simulink library "carnot"  (R2013b)
settings: Solver=ode45  StartTime=0.0  StopTime=10.0  RelTol=1e-3
undefined symbols (not defined in the file or in its folder): A, acol, Ahabit, Awin, Azimuth_Angle, AziWin, B, C, c1, c4, capc, caph, CarnotCallbacks_Density, CarnotCallbacks_Enthalpy, CarnotCallbacks_Enthalpy2Temperature, CarnotCallbacks_Entropy, CarnotCallbacks_Evaporation_Enthalpy, CarnotCallbacks_GlobalMessageLevel, CarnotCallbacks_Grashof, CarnotCallbacks_Heat_Capacity, CarnotCallbacks_Kinematic_Viscosity, CarnotCallbacks_Prandtl, CarnotCallbacks_Saturation_Property, CarnotCallbacks_Saturation_Temperature, CarnotCallbacks_Saturation_Value_Water, CarnotCallbacks_Specific_Volume, CarnotCallbacks_Thermal_Conductivity, CarnotCallbacks_Vapour_Content, CarnotCallbacks_Vapour_Pressure, con, cond, d, Dd, density, dfin, dia, DiameterLastPiece, DPConstant, dpipe, DPLinear, DPQuadratic, emission_out, fluid, FluidMix, FluidType, FPC, frame, g, GeodeticHeight, Gwin, heat_capacity, hgt, HP, Hroom, ID, inlet, K, l, lin, lpipe ... (+29)
undefined symbols (not defined in the file): c2, c3, c5, c6, cwall, dactive, height, mc, mID, rho, tau, UAneighbour, UAwall, uloss
libraries: carnot x333, simulink x25, simulink_extras x7
(part 10 of 16)

== system carnot/Basic/Thermal_Models/sfun_storage_heatexchanger ==
  Tnodes : Inport
  THBin : Inport  Port=2
  Bus Selector : BusSelector  OutputSignals=Temperature,MassFlow,Pressure,FluidType,FluidMix
  Mux1 : Mux  Inputs=5
  storeHX : S-Function  FunctionName=storage_heatexchanger  Parameters=id, nodes, inlet, outlet, pp(1), pp(2), pp(3), pp(4), pp(5), pp(6), pp(7)  EnableBusSupport=off
  Qnodes : Outport
  Thx : Outport  Port=2
  wires:
  Mux1/1 -> storeHX/2
  Bus Selector/5 -> Mux1/5  "<FluidMix>"
  Bus Selector/4 -> Mux1/4  "<FluidType>"
  Bus Selector/3 -> Mux1/3  "<Pressure>"
  Bus Selector/2 -> Mux1/2  "<MassFlow>"
  Bus Selector/1 -> Mux1/1  "<Temperature>"
  Tnodes/1 -> storeHX/1
  storeHX/1 -> Qnodes/1
  THBin/1 -> Bus Selector/1
  storeHX/2 -> Thx/1

== system carnot/Basic/Ventilation/Window_Ventilation ==
  Troom : Inport
  Tamb : Inport  Port=2
  control : Inport  Port=3
  Mux : Mux  Inputs=3
  S-Function : S-Function  FunctionName=tiltvent  Parameters=alpha, H, W  EnableBusSupport=off
  V_rate [m^3/s] : Outport
  wires:
  Tamb/1 -> Mux/2
  control/1 -> Mux/3
  S-Function/1 -> V_rate [m^3/s]/1
  Mux/1 -> S-Function/1
  Troom/1 -> Mux/1

== system carnot/Basic/Weather_and_Sun/Cloudage ==
  Iglob : Inport
  S : Constant  Value=latitude
  S-Function : S-Function  FunctionName=metcloud_s  Parameters=skytype  EnableBusSupport=off
  S1 : Constant  Value=longitude
  S2 : Constant  Value=longitude0
  mux5 : Mux
  cloudage : Outport
  wires:
  S1/1 -> mux5/3
  S/1 -> mux5/2
  mux5/1 -> S-Function/1
  S2/1 -> mux5/4
  S-Function/1 -> cloudage/1
  Iglob/1 -> mux5/1

== system carnot/Basic/Weather_and_Sun/Radiation_Divison ==
  Iglob : Inport
  Demux5 : Demux  Outputs=5
  S : Constant  Value=latitude
  S-Function : S-Function  FunctionName=metrad_s  EnableBusSupport=off
  S1 : Constant  Value=longitude
  S2 : Constant  Value=longitude0
  mux5 : Mux
  Idir : Outport
  Idfu : Outport  Port=2
  SunAngle : Outport  Port=3
  Zenith : Outport  Port=4
  Azimuth : Outport  Port=5
  wires:
  Demux5/5 -> Azimuth/1
  Demux5/4 -> Zenith/1
  Demux5/3 -> SunAngle/1
  Demux5/2 -> Idfu/1
  Demux5/1 -> Idir/1
  S-Function/1 -> Demux5/1
  mux5/1 -> S-Function/1
  Iglob/1 -> mux5/1
  S/1 -> mux5/2
  S1/1 -> mux5/3
  S2/1 -> mux5/4

== system carnot/Basic/Weather_and_Sun/Sky_Temperature ==
  Tamb : Inport
  hum : Inport  Port=2
  cloudage : Inport  Port=3
  S-Function : S-Function  FunctionName=metsky_s  Parameters=tskymodel  EnableBusSupport=off
  mux6 : Mux  Inputs=3
  Tsky : Outport
  wires:
  S-Function/1 -> Tsky/1
  mux6/1 -> S-Function/1
  Tamb/1 -> mux6/1
  hum/1 -> mux6/2
  cloudage/1 -> mux6/3

== system carnot/Basic/Weather_and_Sun/Solar_Declination_Angle ==
  time : Inport
  S-Function : S-Function  FunctionName=solardeclination  EnableBusSupport=off
  declination : Outport
  wires:
  time/1 -> S-Function/1
  S-Function/1 -> declination/1

== system carnot/Basic/Weather_and_Sun/Solar_Extraterrestrial_Radiation ==
  time : Inport
  S-Function : S-Function  FunctionName=solarextraterrestrialradiaton  EnableBusSupport=off
  I_extra : Outport
  wires:
  S-Function/1 -> I_extra/1
  time/1 -> S-Function/1

== system carnot/Basic/Weather_and_Sun/Solar_Hour_Angle ==
  note: hourangle = (true_solar_time - 12*3600)*2*pi/24/3600
  time : Inport
  2*pi/(24*3600) : Gain  Gain=2*pi/(24*3600)
  Add : Sum  Inputs=+-
  Constant : Constant  Value=12*3600
  S-Function : S-Function  FunctionName=solartime  Parameters=timezone, longitude  EnableBusSupport=off
  solar_hour_angle : Outport
  wires:
  time/1 -> S-Function/1
  S-Function/1 -> Add/1
  Add/1 -> 2*pi/(24*3600)/1
  2*pi/(24*3600)/1 -> solar_hour_angle/1
  Constant/1 -> Add/2

== system carnot/Basic/Weather_and_Sun/Solar_Position ==
  Solar_Position : S-Function  FunctionName=sunpos  Parameters=longi lati timezone  EnableBusSupport=off
  Out1 : Outport
  wires:
  Solar_Position/1 -> Out1/1

== system carnot/Basic/Weather_and_Sun/Solar_Time ==
  time : Inport
  S-Function : S-Function  FunctionName=solartime  Parameters=timezone, longitude  EnableBusSupport=off
  solartime : Outport
  wires:
  S-Function/1 -> solartime/1
  time/1 -> S-Function/1

== system carnot/Basic/Weather_and_Sun/WDB_Creator ==
  TimeValueComment : Inport
  Zenith_Angle : Inport  Port=2
  Azimuth_Angle : Inport  Port=3
  Solar_Radiation_beam_normal : Inport  Port=4
  Solar_Radiation_diffuse_horizontal : Inport  Port=5
  Temperature_Ambient : Inport  Port=6
  Temperature_Sky_Radiation : Inport  Port=7
  Relative_Humidity : Inport  Port=8
  Precipitation : Inport  Port=9
  Cloud_Index : Inport  Port=10
  Station_Pressure : Inport  Port=11
  Wind_Speed : Inport  Port=12
  Wind_Direction : Inport  Port=13
  Incidence_Angle_sun : Inport  Port=14
  Incidence_Angle_longitudinal : Inport  Port=15
  Incidence_Angle_transversal : Inport  Port=16
  Solar_Radiation_direct_surface : Inport  Port=17
  Solar_Radiation_diffuse_surface : Inport  Port=18
  Bus Creator : BusCreator  InitFcn=load WDB.mat  Inputs=18  OutDataTypeStr=Bus: WDB
  WDB : Outport
  wires:
  Bus Creator/1 -> WDB/1  "WDB"
  Solar_Radiation_diffuse_surface/1 -> Bus Creator/18  "Solar_Radiation_diffuse_surface"
  Solar_Radiation_direct_surface/1 -> Bus Creator/17  "Solar_Radiation_direct_surface"
  Incidence_Angle_transversal/1 -> Bus Creator/16  "Incidence_Angle_transversal"
  Incidence_Angle_longitudinal/1 -> Bus Creator/15  "Incidence_Angle_longitudinal"
  Incidence_Angle_sun/1 -> Bus Creator/14  "Incidence_Angle_sun"
  Wind_Direction/1 -> Bus Creator/13  "Wind_Direction"
  Wind_Speed/1 -> Bus Creator/12  "Wind_Speed"
  Station_Pressure/1 -> Bus Creator/11  "Station_Pressure"
  Cloud_Index/1 -> Bus Creator/10  "Cloud_Index"
  Precipitation/1 -> Bus Creator/9  "Precipitation"
  Relative_Humidity/1 -> Bus Creator/8  "Relative_Humidity"
  Temperature_Sky_Radiation/1 -> Bus Creator/7  "Temperature_Sky_Radiation"
  Temperature_Ambient/1 -> Bus Creator/6  "Temperature_Ambient"
  Solar_Radiation_diffuse_horizontal/1 -> Bus Creator/5  "Solar_Radiation_diffuse_horizontal"
  Azimuth_Angle/1 -> Bus Creator/3  "Azimuth_Angle"
  Zenith_Angle/1 -> Bus Creator/2  "Zenith_Angle"
  TimeValueComment/1 -> Bus Creator/1  "TimeValueComment"
  Solar_Radiation_beam_normal/1 -> Bus Creator/4  "Solar_Radiation_beam_normal"

== system carnot/Hydraulics/Flow_Diverter/Subsystem ==
  In1 : Inport
  Bus Selector10 : BusSelector  OutputSignals=MassFlow,DPConstant,DPLinear,DPQuadratic
  Mux : Mux
  Out1 : Outport
  wires:
  Mux/1 -> Out1/1
  In1/1 -> Bus Selector10/1
  Bus Selector10/4 -> Mux/4  "<DPQuadratic>"
  Bus Selector10/3 -> Mux/3  "<DPLinear>"
  Bus Selector10/2 -> Mux/2  "<DPConstant>"
  Bus Selector10/1 -> Mux/1  "<MassFlow>"

== system carnot/Hydraulics/Flow_Diverter/increase_ID ==
  In1 : Inport
  Abs : Abs
  Bias : Bias  Bias=1
  Dot Product1 : DotProduct  InputSameDT=on  OutDataTypeStr=Inherit: Inherit via internal rule
  Sign : Signum
  Out1 : Outport
  wires:
  In1/1 -> Abs/1, Sign/1
  Dot Product1/1 -> Out1/1
  Abs/1 -> Bias/1
  Sign/1 -> Dot Product1/1
  Bias/1 -> Dot Product1/2

== system carnot/Hydraulics/Flow_Mixer/PT1_for_fdiv ==
  ID_1 : Inport
  ID_2 : Inport  Port=2
  fdiv : Inport  Port=3
  Compare To Zero : simulink/Logic and Bit Operations/Compare To Zero  relop=<=  OutDataTypeStr=uint8
  Compare To Zero1 : simulink/Logic and Bit Operations/Compare To Zero  relop=<=  OutDataTypeStr=uint8
  Constant : Constant  Value=0
  Constant1 : Constant
  Gain1 : Gain  Gain=2
  Index Vector : MultiPortSwitch  DataPortOrder=Zero-based contiguous  zeroidx=on
  MinMax2 : MinMax  Function=max  Inputs=2
  Transfer Fcn (with initial states) : simulink_extras/Additional Linear/Transfer Fcn (with initial states)  N=[1]  D="[t  1]"  X0=0.5
  f_div : Outport
  wires:
  Index Vector/1 -> f_div/1
  Gain1/1 -> MinMax2/2
  Constant1/1 -> Index Vector/4
  Transfer Fcn (with initial states)/1 -> Index Vector/2
  Constant/1 -> Index Vector/3
  ID_2/1 -> Compare To Zero1/1
  ID_1/1 -> Compare To Zero/1
  MinMax2/1 -> Index Vector/1
  Compare To Zero/1 -> MinMax2/1
  Compare To Zero1/1 -> Gain1/1
  fdiv/1 -> Transfer Fcn (with initial states)/1

== system carnot/Hydraulics/Flow_Mixer_Thermostatic/Icontrol_fdiv ==
  ID_1 : Inport
  ID_2 : Inport  Port=2
  Twarm : Inport  Port=3
  Tset : Inport  Port=4
  Compare To Zero : simulink/Logic and Bit Operations/Compare To Zero  relop=<=  OutDataTypeStr=uint8
  Compare To Zero1 : simulink/Logic and Bit Operations/Compare To Zero  relop=<=  OutDataTypeStr=uint8
  Constant : Constant  Value=0
  Constant1 : Constant
  Gain : Gain  Gain=t1  SaturateOnIntegerOverflow=on  OutDataTypeStr=Inherit: Same as input  ParamDataTypeStr=Inherit: Same as input
  Gain1 : Gain  Gain=2
  Index Vector : MultiPortSwitch  DataPortOrder=Zero-based contiguous  zeroidx=on
  Integrator : Integrator  LimitOutput=on  UpperSaturationLimit=1  LowerSaturationLimit=0
  MinMax2 : MinMax  Function=max  Inputs=2
  diff_T : Sum  Inputs=-+  SaturateOnIntegerOverflow=on  InputSameDT=on  OutDataTypeStr=Inherit: Same as first input
  f_div : Outport
  wires:
  diff_T/1 -> Gain/1
  Gain/1 -> Integrator/1
  Twarm/1 -> diff_T/1
  Tset/1 -> diff_T/2
  Index Vector/1 -> f_div/1
  Gain1/1 -> MinMax2/2
  Constant1/1 -> Index Vector/4
  Integrator/1 -> Index Vector/2
  Constant/1 -> Index Vector/3
  ID_2/1 -> Compare To Zero1/1
  ID_1/1 -> Compare To Zero/1
  MinMax2/1 -> Index Vector/1
  Compare To Zero/1 -> MinMax2/1
  Compare To Zero1/1 -> Gain1/1

== system carnot/Hydraulics/Valve_ThermoTset/thermostat charcteristic ==
  T : Inport
  Tset : Inport  Port=2
  Backlash : Backlash  BacklashWidth=bl
  Bias : Bias  Bias=op
  Bias1 : Bias  Bias=bl/2
  Gain : Gain  Gain=op/(p-bl)
  Saturation : Saturate  UpperLimit=1  LowerLimit=0
  Sensor : TransferFcn  Denominator=[ts 1]
  Sum1 : Sum  Inputs=-+  SaturateOnIntegerOverflow=on  InputSameDT=on  OutDataTypeStr=Inherit: Same as first input
  pos : Outport  InitialOutput=0
  wires:
  Tset/1 -> Sum1/2
  T/1 -> Sensor/1
  Bias/1 -> Saturation/1
  Saturation/1 -> pos/1
  Sum1/1 -> Bias1/1
  Backlash/1 -> Gain/1
  Gain/1 -> Bias/1
  Bias1/1 -> Backlash/1
  Sensor/1 -> Sum1/1

== system carnot/Load/General/Load_Data_Button ==

== system carnot/Load/General/Load_from_File ==
  Constant : Constant
  From_Workspace : FromWorkspace  VariableName=DE_ElectricLoad_SFH_try04_VDI4655  SampleTime=0
  Terminator : Terminator
  Unit Delay : UnitDelay  SampleTime=t_sample
  Out1 : Outport
  wires:
  Unit Delay/1 -> Terminator/1
  Constant/1 -> Unit Delay/1
  From_Workspace/1 -> Out1/1

== system carnot/Load/General/Repeating_Profile ==
  Add : Sum  Inputs=1
  Pulse Generator : DiscretePulseGenerator  PulseType=Time based  Amplitude=rep_seq_y  Period=period  PulseWidth=rep_seq_d*100/period  PhaseDelay=rep_seq_t
  Out1 : Outport
  wires:
  Add/1 -> Out1/1
  Pulse Generator/1 -> Add/1

== system carnot/Load/Hot_Water_Tapping/Applications ==
  Hot_Water_Consumption_EN13203 : Subsystem
      mask Display: plot(0,0,140,130,[70,76,78,63,65,70,70,10],[80,78,74,74,78,80,100,100],[23,23,20,10],[43,47,50,50],[10,10,20,28,30,10],[30,20,20,23,30,30],[22,17],[54,54],[20,20],[54,50],[90,90,50,50],[10,-0,-0,10],[63,64],[60,72],[61,62],[38,50],[60,61],[13,27],[90,85,81,76,70,65,59,54,50],[6,4,6,4,6,4,5,3,5],[68,69],[56,68],[68,68],[32,44],[67,67],[13,23],[73,73],[61,71],[73,73],[43,52],[74,73],[21,36],[78,77],[56,67],[79,79],[34,45],[78,77],[9,23],[82,81],[14,26])
  Hot_Water_Consumption_basic : Subsystem
      mask Display: plot(0,0,140,130,[70,76,78,63,65,70,70,10],[80,78,74,74,78,80,100,100],[23,23,20,10],[43,47,50,50],[10,10,20,28,30,10],[30,20,20,23,30,30],[22,17],[54,54],[20,20],[54,50],[90,90,50,50],[10,-0,-0,10],[63,64],[60,72],[61,62],[38,50],[60,61],[13,27],[90,85,81,76,70,65,59,54,50],[6,4,6,4,6,4,5,3,5],[68,69],[56,68],[68,68],[32,44],[67,67],[13,23],[73,73],[61,71],[73,73],[43,52],[74,73],[21,36],[78,77],[56,67],[79,79],[34,45],[78,77],[9,23],[82,81],[14,26])

== system carnot/Load/Hot_Water_Tapping/DHW_Energy_Tapping ==
  Tc : Inport
  Rate Transition : RateTransition
  Rate Transition1 : RateTransition
  s_function : S-Function  FunctionName=dhw_EN13203  Parameters=times,energies,coeffs,dT_set,mdot_nom  EnableBusSupport=off
  mdot : Outport
  Tset : Outport  Port=2
  wires:
  Rate Transition1/1 -> Tset/1
  Rate Transition/1 -> mdot/1
  Tc/1 -> s_function/1
  s_function/1 -> Rate Transition/1
  s_function/2 -> Rate Transition1/1

== system carnot/Load/Hot_Water_Tapping/EU_Tapping_Cycle ==
  Tc : Inport
  DHW_Energy_Tapping : carnot/Load/Hot_Water_Tapping/DHW_Energy_Tapping  mdot_nom=1  times=times  energies=energies  dT_set=dT_set  coeffs=mdot
  mdot : Outport
  Tset : Outport  Port=2
  wires:
  Tc/1 -> DHW_Energy_Tapping/1
  DHW_Energy_Tapping/2 -> Tset/1
  DHW_Energy_Tapping/1 -> mdot/1

== system carnot/Load/Hot_Water_Tapping/T_cold_Water_Location ==
  Sine Wave : Sin  Amplitude=Tamp  Bias=T  Frequency=(2*pi/365/24/3600)  Phase=(2*pi*dshift/365)  SampleTime=0
  Tc : Outport  InitialOutput=0
  wires:
  Sine Wave/1 -> Tc/1

== system carnot/Load/Hot_Water_Tapping/T_cold_Water_Season ==
  S-Function : S-Function  FunctionName=season_temperature  Parameters=month1 temp1 month2 temp2 form  EnableBusSupport=off
  Tc : Outport
  wires:
  S-Function/1 -> Tc/1

== system carnot/Load/Hot_Water_Tapping/T_cold_Water_Sine ==
  Sine Wave : Sin  Amplitude=Tamp  Bias=T  Frequency=(2*pi/365/24/3600)  Phase=(2*pi*dshift/365)  SampleTime=0
  Tc : Outport  InitialOutput=0
  wires:
  Sine Wave/1 -> Tc/1

== system carnot/Load/Hot_Water_Tapping/Water_Tap ==
  mdot : Inport
  Tc : Inport  Port=2
  basic_create_THB : carnot/Basic/Hydraulics/basic_create_THB  p=p  fluid=fluid  mix=mix  dia=dia  hgt=0  mID=1
  THB : Outport
  wires:
  mdot/1 -> basic_create_THB/1
  Tc/1 -> basic_create_THB/2
  basic_create_THB/1 -> THB/1

== system carnot/Load/Hot_Water_Tapping/create_mdot ==
  note: Don't change any names
      | in this subsystem!
  Gain : Gain  Gain=1/10000  SaturateOnIntegerOverflow=on  OutDataTypeStr=Inherit: Same as input  ParamDataTypeStr=Inherit: Same as input
  Multiport Switch : MultiPortSwitch  Inputs=2  SaturateOnIntegerOverflow=on  InputSameDT=on
  Product : Product  Inputs=3  SaturateOnIntegerOverflow=on  InputSameDT=on  OutDataTypeStr=Inherit: Same as first input
  RS Month : simulink/Sources/Repeating Sequence  rep_seq_t=[0 2678399 2678399 5097599 5097599 7775999 7775999 10367999 10367999 13046399 13046399 15638399 15638399 18316799 18316799 20995199 20995199 23587199 23587199 26265599 26265599 28857599 28857599 31536000]  rep_seq_y=[99 99 97 97 100 100 100 100 103 103 105 105 109 109 112 112 108 108 105 105 101 101 100 100]
  RS Sunday : simulink/Sources/Repeating Sequence  rep_seq_t="100*[0 18 18 36 36 54 54 72 72 90 90 108 108 126 126 144 144 162 162 180 180 198 198 216 216 234 234 252 252 270 270 288 288 306 306 324 324 342 342 360 360 378 378 396 396 414 414 432 432 450 450 468 468 486 486 504 504 522 522 540 540 558 558 576 576 594 594 612 612 630 630 648 648 666 666 684 684 702 702 720 720 738 738 756 756 774 774 792 792 810 810 828 828 846 846  864]"  rep_seq_y=[0 0 0 0 0.5 0.5 0.5 0.5 0.5 0.5 0.5 0.5 1 1 1 1 1 1 1 1 1 1 1 1 1 1 2 2 2 2 3 3 2 2 2 2 2 2 2 2 3 3 2 2 2 2 2 2 3 3 3 3 3 3 3 3 3 3 2 2 2 2 1 1 1 1 2 2 2 2 3 3 3 3 3 3 3 3 2 2 2 2 2 2 2 2 2 2 1 1 1 1 1 1 1 1]
  RS Weekday : simulink/Sources/Repeating Sequence  rep_seq_t="100*[0 18 18 36 36 54 54 72 72 90 90 108 108 126 126 144 144 162 162 180 180 198 198 216 216 234 234 252 252 270 270 288 288 306 306 324 324 342 342 360 360 378 378 396 396 414 414 432 432 450 450 468 468 486 486 504 504 522 522 540 540 558 558 576 576 594 594 612 612 630 630 648 648 666 666 684 684 702 702 720 720 738 738 756 756 774 774 792 792 810 810 828 828 846 846  864]"  rep_seq_y=[0.5 0.5 0.5 0.5 0.5 0.5 0.5 0.5 0.5 0.5 0.5 0.5 1 1 1 1 1 1 1 1 2 2 2 2 3 3 3 3 5 5 5 5 5 5 5 5 4 4 4 4 3 3 2 2 2 2 2 2 3 3 3 3 4 4 4 4 3 3 2 2 2 2 1 1 1 1 2 2 2 2 3 3 3 3 3 3 3 3 2 2 2 2 2 2 2 2 2 2 1 1 1 1 1 1 1 1]
  Repeating Sequence Day of the Week : simulink/Sources/Repeating Sequence  rep_seq_t=[0 5*24*3600 5*24*3600 7*24*3600]  rep_seq_y=[1 1 2 2]
  mdot0 : Constant  Value=0.1
  mdot : Outport
  wires:
  RS Month/1 -> Product/2
  RS Weekday/1 -> Multiport Switch/2
  Gain/1 -> mdot/1
  Product/1 -> Gain/1
  mdot0/1 -> Product/1
  Multiport Switch/1 -> Product/3
  RS Sunday/1 -> Multiport Switch/3
  Repeating Sequence Day of the Week/1 -> Multiport Switch/1

== system carnot/Load/Hot_Water_Tapping/mdot_40_20_40 ==
  Add : Sum  Inputs=1
  Pulse Generator : DiscretePulseGenerator  PulseType=Time based  Amplitude=rep_seq_y  Period=period  PulseWidth=rep_seq_d*100/period  PhaseDelay=rep_seq_t
  Out1 : Outport
  wires:
  Pulse Generator/1 -> Add/1
  Add/1 -> Out1/1

== system carnot/Load/Hot_Water_Tapping/mdot_DHWcalc ==
  dhw_from_Workspace : FromWorkspace  VariableName=DHW0001_DHW  SampleTime=0  OutputAfterFinalValue=Setting to zero
  to kg_s : Gain  Gain=1/3600
  mdot : Outport
  wires:
  dhw_from_Workspace/1 -> to kg_s/1
  to kg_s/1 -> mdot/1

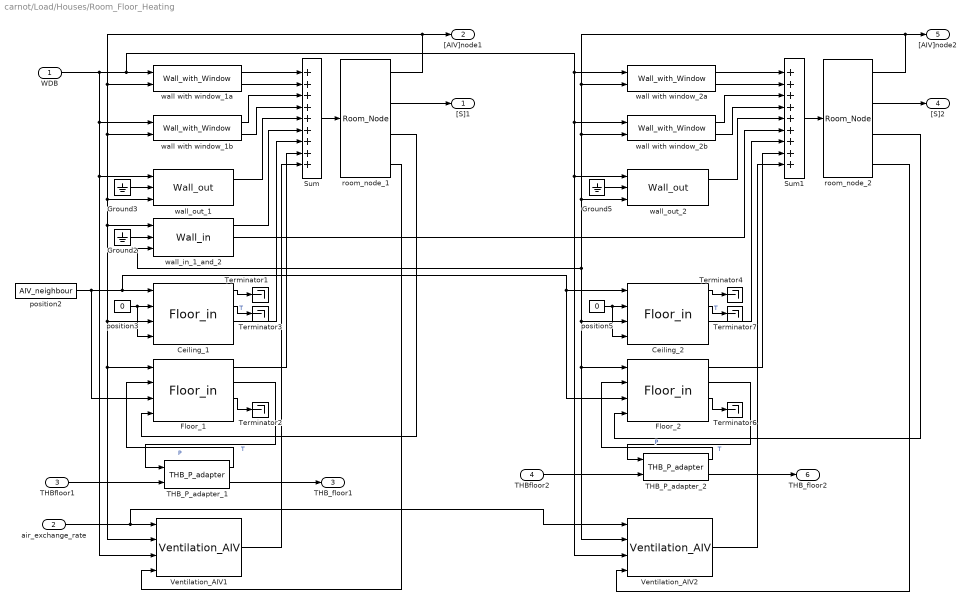
== system carnot/Load/Houses/Room_Floor_Heating ==
  WDB : Inport
  air_exchange_rate : Inport  Port=2
  THBfloor1 : Inport  Port=3
  THBfloor2 : Inport  Port=4
  Ceiling_1 : carnot/Load/Houses/wall_floor/Floor_in  wallsize=[5 5]  t0=20  d=[0.015 0.38 0.02]  cond=[1.4 0.79 0.7]  cwall=[0.28 0.28 0.28]*3600  rho=[2000 1800 1400]  misc=[.65 .65]  dactive=-1  tau=1000*3600
  Ceiling_2 : carnot/Load/Houses/wall_floor/Floor_in  wallsize=[5 5]  t0=20  d=[0.015 0.38 0.02]  cond=[1.4 0.79 0.7]  cwall=[0.28 0.28 0.28]*3600  rho=[2000 1800 1400]  misc=[.65 .65]  dactive=-1  tau=1000*3600
  Floor_1 : carnot/Load/Houses/wall_floor/Floor_in  wallsize=[5 5]  t0=20  d=[0.015 0.38 0.02]  cond=[1.4 0.79 0.7]  cwall=[0.28 0.28 0.28]*3600  rho=[2000 1800 1400]  misc=[.65 .65]  dactive=0.02  tau=1000*3600
  Floor_2 : carnot/Load/Houses/wall_floor/Floor_in  wallsize=[5 5]  t0=20  d=[0.015 0.38 0.02]  cond=[1.4 0.79 0.7]  cwall=[0.28 0.28 0.28]*3600  rho=[2000 1800 1400]  misc=[.65 .65]  dactive=0.02  tau=1000*3600
  Ground2 : Ground
  Ground3 : Ground
  Ground5 : Ground
  Sum : Sum  Inputs=9  SaturateOnIntegerOverflow=on  InputSameDT=on  OutDataTypeStr=Inherit: Same as first input
  Sum1 : Sum  Inputs=9  SaturateOnIntegerOverflow=on  InputSameDT=on  OutDataTypeStr=Inherit: Same as first input
  THB_P_adapter_1 : carnot/Load/Houses/ventilation_heating/THB_P_adapter  mass=1  ua=800*5*5/0.2*0.022*3.1415  t0=20
  THB_P_adapter_2 : carnot/Load/Houses/ventilation_heating/THB_P_adapter  mass=1  ua=800*5*5/0.2*0.022*3.1415  t0=20
  Terminator{1..4,6..7} (6 alike) : Terminator
  Ventilation_AIV1 : carnot/Source/Ventilation/Ventilation_AIV  co2=400
  Ventilation_AIV2 : carnot/Source/Ventilation/Ventilation_AIV  co2=400
  position2 : Constant  Value=AIV_neighbour
  position3 : Constant  Value=0
  position5 : Constant  Value=0
  room_node_1 : carnot/Load/Houses/room_node/Room_Node  zoneairvolume=5*5*2.5  zoneheight=2.5  zonestartTEMP=20  zonestartWATER=55  timeconst=100  heatperfect=natural  lookuptime=[0 24]*3600  lookupvalue=[20 20]  AirPressure=101300
  room_node_2 : carnot/Load/Houses/room_node/Room_Node  zoneairvolume=5*5*2.5  zoneheight=2.5  zonestartTEMP=20  zonestartWATER=55  timeconst=100  heatperfect=natural  lookuptime=[0 24]*3600  lookupvalue=[20 20]  AirPressure=101300
  wall with window_1a : carnot/Load/Houses/wall_floor/Wall_with_Window  wallsize=[2.5 5]  windowsize=[1 2]  frame=0.1  pos=90  t0=20  tau=1000*3600  g=0.7
  wall with window_1b : carnot/Load/Houses/wall_floor/Wall_with_Window  wallsize=[2.5 5]  windowsize=[1 2]  frame=0.1  pos=0  t0=20  tau=1000*3600  g=0.7
  wall with window_2a : carnot/Load/Houses/wall_floor/Wall_with_Window  wallsize=[2.5 5]  windowsize=[1 2]  frame=0.1  pos=-90  t0=20  tau=1000*3600  g=0.7
  wall with window_2b : carnot/Load/Houses/wall_floor/Wall_with_Window  wallsize=[2.5 5]  windowsize=[1 2]  frame=0.1  pos=0  t0=20  tau=1000*3600  g=0.7
  wall_in_1_and_2 : carnot/Load/Houses/wall_floor/Wall_in  wallsize=[2.5 5]  d=[0.015 0.38 0.02]  cond=[1.4 0.79 0.7]  cwall=[0.28 0.28 0.28]*3600  rho=[2000 1800 1400]  emission_in=.96  dactive=-1  t0=20  tau=1000*3600
  wall_out_1 : carnot/Load/Houses/wall_floor/Wall_out  wallsize=[2.5 5]  pos=180  t0=20  d=[0.1 0.38]  cond=[0.04 0.79]  cwall=[0.28 0.28]*3600  rho=[900 1800]  reflectground=0.2  abs_emiss=[0.65 0.97 0.96]  tau=1000*3600  dactive=-1
  wall_out_2 : carnot/Load/Houses/wall_floor/Wall_out  wallsize=[2.5 5]  pos=180  t0=20  d=[0.1 0.38]  cond=[0.04 0.79]  cwall=[0.28 0.28]*3600  rho=[900 1800]  reflectground=0.2  abs_emiss=[0.65 0.97 0.96]  tau=1000*3600  dactive=-1
  "[S]1" : Outport
  "[AIV]node1" : Outport  Port=2
  THB_floor1 : Outport  Port=3
  "[S]2" : Outport  Port=4
  "[AIV]node2" : Outport  Port=5
  THB_floor2 : Outport  Port=6
  wires:
  wall_in_1_and_2/1 -> Sum/6
  WDB/1 -> wall with window_1b/1, wall_out_1/1, Ventilation_AIV1/3, wall with window_1a/1, wall_out_2/1, Ventilation_AIV2/3, wall with window_2b/1, wall with window_2a/1
  wall with window_1a/1 -> Sum/1
  wall with window_1a/2 -> Sum/2
  wall with window_1b/1 -> Sum/3
  wall_out_1/1 -> Sum/5
  wall with window_1b/2 -> Sum/4
  room_node_1/2 -> "[S]1"/1
  Ceiling_1/1 -> Terminator1/1
  Ceiling_1/2 -> Terminator3/1  "T"
  Floor_1/3 -> Terminator2/1
  position3/1 -> Ceiling_1/2, Ceiling_1/4
  Floor_1/1 -> Sum/8
  Ceiling_1/3 -> Sum/7
  Ventilation_AIV1/1 -> Sum/9
  THBfloor1/1 -> THB_P_adapter_1/2
  Floor_1/2 -> THB_P_adapter_1/1  "T"
  THB_P_adapter_1/1 -> Floor_1/2  "P"
  THB_P_adapter_1/2 -> THB_floor1/1
  room_node_1/4 -> Ventilation_AIV1/4
  room_node_1/3 -> Floor_1/4
  Ground2/1 -> wall_in_1_and_2/2
  Ground3/1 -> wall_out_1/2
  position2/1 -> Floor_1/3, Ceiling_1/1, Ceiling_2/1, Floor_2/3
  wall with window_2a/1 -> Sum1/1
  wall with window_2a/2 -> Sum1/2
  wall with window_2b/1 -> Sum1/3
  wall_out_2/1 -> Sum1/5
  wall with window_2b/2 -> Sum1/4
  room_node_2/2 -> "[S]2"/1
  Ceiling_2/1 -> Terminator4/1
  Ceiling_2/2 -> Terminator7/1  "T"
  Floor_2/3 -> Terminator6/1
  position5/1 -> Ceiling_2/4, Ceiling_2/2
  Floor_2/1 -> Sum1/8
  Ceiling_2/3 -> Sum1/7
  Ventilation_AIV2/1 -> Sum1/9
  THBfloor2/1 -> THB_P_adapter_2/2
  Floor_2/2 -> THB_P_adapter_2/1  "T"
  THB_P_adapter_2/1 -> Floor_2/2  "P"
  THB_P_adapter_2/2 -> THB_floor2/1
  room_node_2/4 -> Ventilation_AIV2/4
  room_node_2/3 -> Floor_2/4
  Ground5/1 -> wall_out_2/2
  wall_in_1_and_2/2 -> Sum1/6
  air_exchange_rate/1 -> Ventilation_AIV2/1, Ventilation_AIV1/1
  room_node_1/1 -> wall with window_1a/2, wall with window_1b/2, wall_in_1_and_2/1, Ceiling_1/3, Floor_1/1, Ventilation_AIV1/2, wall_out_1/3, "[AIV]node1"/1
  room_node_2/1 -> wall_out_2/3, Floor_2/1, Ventilation_AIV2/2, Ceiling_2/3, wall_in_1_and_2/3, wall with window_2b/2, wall with window_2a/2, "[AIV]node2"/1
  Sum/1 -> room_node_1/1
  Sum1/1 -> room_node_2/1

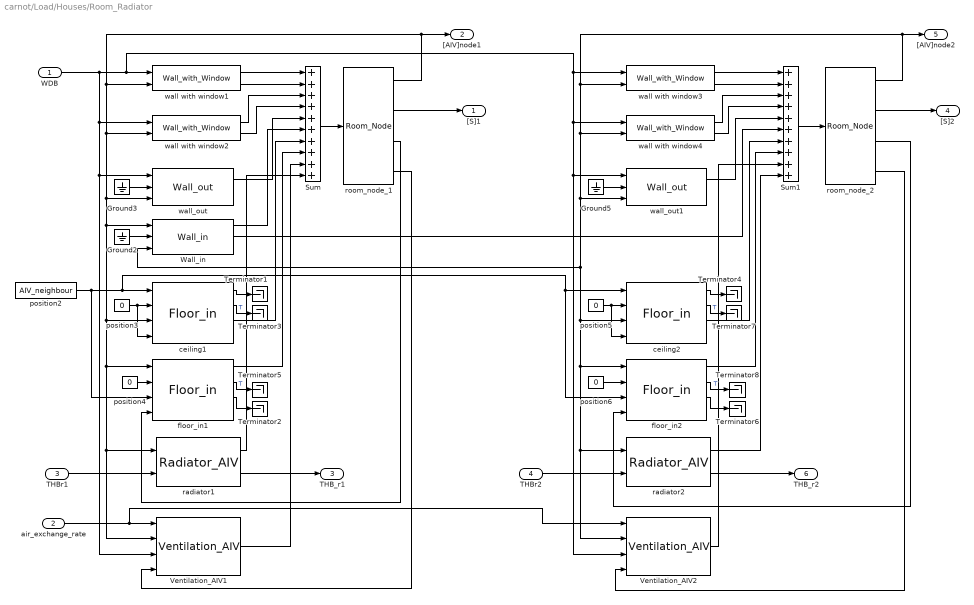
== system carnot/Load/Houses/Room_Radiator ==
  WDB : Inport
  air_exchange_rate : Inport  Port=2
  THBr1 : Inport  Port=3
  THBr2 : Inport  Port=4
  Ground2 : Ground
  Ground3 : Ground
  Ground5 : Ground
  Sum : Sum  Inputs=10  SaturateOnIntegerOverflow=on  InputSameDT=on  OutDataTypeStr=Inherit: Same as first input
  Sum1 : Sum  Inputs=10  SaturateOnIntegerOverflow=on  InputSameDT=on  OutDataTypeStr=Inherit: Same as first input
  Terminator{1..8} (8 alike) : Terminator
  Ventilation_AIV1 : carnot/Source/Ventilation/Ventilation_AIV  co2=400
  Ventilation_AIV2 : carnot/Source/Ventilation/Ventilation_AIV  co2=400
  Wall_in : carnot/Load/Houses/wall_floor/Wall_in  wallsize=[2.5 5]  d=[0.015 0.38 0.02]  cond=[1.4 0.79 0.7]  cwall=[0.28 0.28 0.28]*3600  rho=[2000 1800 1400]  emission_in=0.96  dactive=-1  t0=20  tau=1000*3600
  ceiling1 : carnot/Load/Houses/wall_floor/Floor_in  wallsize=[5 5]  t0=20  d=[0.015 0.38 0.02]  cond=[1.4 0.79 0.7]  cwall=[0.28 0.28 0.28]*3600  rho=[2000 1800 1400]  misc=[.65 .65]  dactive=-1  tau=1000*3600
  ceiling2 : carnot/Load/Houses/wall_floor/Floor_in  wallsize=[5 5]  t0=20  d=[0.015 0.38 0.02]  cond=[1.4 0.79 0.7]  cwall=[0.28 0.28 0.28]*3600  rho=[2000 1800 1400]  misc=[.65 .65]  dactive=-1  tau=1000*3600
  floor_in1 : carnot/Load/Houses/wall_floor/Floor_in  wallsize=[5 5]  t0=20  d=[0.015 0.38 0.02]  cond=[1.4 0.79 0.7]  cwall=[0.28 0.28 0.28]*3600  rho=[2000 1800 1400]  misc=[.65 .65]  dactive=-1  tau=1000*3600
  floor_in2 : carnot/Load/Houses/wall_floor/Floor_in  wallsize=[5 5]  t0=20  d=[0.015 0.38 0.02]  cond=[1.4 0.79 0.7]  cwall=[0.28 0.28 0.28]*3600  rho=[2000 1800 1400]  misc=[.65 .65]  dactive=-1  tau=1000*3600
  position2 : Constant  Value=AIV_neighbour
  position{3..6} (4 alike) : Constant  Value=0
  radiator1 : carnot/Source/Heat_Exchanger/Radiator_AIV  pnom=500  dtnom=40  expo=1.3  mcap=5*4182  ra=0.47  tini=20  lin=0  qua=1000
  radiator2 : carnot/Source/Heat_Exchanger/Radiator_AIV  pnom=500  dtnom=40  expo=1.3  mcap=5*4182  ra=0.47  tini=20  lin=0  qua=1000
  room_node_1 : carnot/Load/Houses/room_node/Room_Node  zoneairvolume=5*5*2.5  zoneheight=2.5  zonestartTEMP=20  zonestartWATER=55  timeconst=100  heatperfect=natural  lookuptime=[0 24]*3600  lookupvalue=[20 20]  AirPressure=101300
  room_node_2 : carnot/Load/Houses/room_node/Room_Node  zoneairvolume=5*5*2.5  zoneheight=2.5  zonestartTEMP=20  zonestartWATER=55  timeconst=100  heatperfect=natural  lookuptime=[0 24]*3600  lookupvalue=[20 20]  AirPressure=101300
  wall with window1 : carnot/Load/Houses/wall_floor/Wall_with_Window  wallsize=[2.5 5]  windowsize=[1 2]  frame=0.1  pos=90  t0=20  tau=1000*3600  g=0.7
  wall with window2 : carnot/Load/Houses/wall_floor/Wall_with_Window  wallsize=[2.5 5]  windowsize=[1 2]  frame=0.1  pos=0  t0=20  tau=1000*3600  g=0.7
  wall with window3 : carnot/Load/Houses/wall_floor/Wall_with_Window  wallsize=[2.5 5]  windowsize=[1 2]  frame=0.1  pos=-90  t0=20  tau=1000*3600  g=0.7
  wall with window4 : carnot/Load/Houses/wall_floor/Wall_with_Window  wallsize=[2.5 5]  windowsize=[1 2]  frame=0.1  pos=0  t0=20  tau=1000*3600  g=0.7
  wall_out : carnot/Load/Houses/wall_floor/Wall_out  wallsize=[2.5 5]  pos=180  t0=20  d=[0.1 0.38]  cond=[0.04 0.79]  cwall=[0.28 0.28]*3600  rho=[900 1800]  reflectground=0.2  abs_emiss=[0.65 0.97 0.96]  tau=1000*3600  dactive=-1
  wall_out1 : carnot/Load/Houses/wall_floor/Wall_out  wallsize=[2.5 5]  pos=180  t0=20  d=[0.1 0.38]  cond=[0.04 0.79]  cwall=[0.28 0.28]*3600  rho=[900 1800]  reflectground=0.2  abs_emiss=[0.65 0.97 0.96]  tau=1000*3600  dactive=-1
  "[S]1" : Outport
  "[AIV]node1" : Outport  Port=2
  THB_r1 : Outport  Port=3
  "[S]2" : Outport  Port=4
  "[AIV]node2" : Outport  Port=5
  THB_r2 : Outport  Port=6
  wires:
  Wall_in/1 -> Sum/6
  WDB/1 -> wall with window2/1, wall_out/1, Ventilation_AIV1/3, wall with window1/1, wall_out1/1, Ventilation_AIV2/3, wall with window4/1, wall with window3/1
  wall with window1/1 -> Sum/1
  wall with window1/2 -> Sum/2
  wall with window2/1 -> Sum/3
  wall_out/1 -> Sum/5
  wall with window2/2 -> Sum/4
  room_node_1/2 -> "[S]1"/1
  ceiling1/1 -> Terminator1/1
  ceiling1/2 -> Terminator3/1  "T"
  floor_in1/3 -> Terminator2/1
  position3/1 -> ceiling1/2, ceiling1/4
  floor_in1/1 -> Sum/8
  ceiling1/3 -> Sum/7
  Ventilation_AIV1/1 -> Sum/9
  THBr1/1 -> radiator1/2
  radiator1/2 -> THB_r1/1
  room_node_1/4 -> Ventilation_AIV1/4
  room_node_1/3 -> floor_in1/4
  Ground2/1 -> Wall_in/2
  Ground3/1 -> wall_out/2
  position2/1 -> floor_in1/3, ceiling1/1, ceiling2/1, floor_in2/3
  wall with window3/1 -> Sum1/1
  wall with window3/2 -> Sum1/2
  wall with window4/1 -> Sum1/3
  wall_out1/1 -> Sum1/5
  wall with window4/2 -> Sum1/4
  room_node_2/2 -> "[S]2"/1
  ceiling2/1 -> Terminator4/1
  ceiling2/2 -> Terminator7/1  "T"
  floor_in2/3 -> Terminator6/1
  position5/1 -> ceiling2/4, ceiling2/2
  floor_in2/1 -> Sum1/8
  ceiling2/3 -> Sum1/7
  Ventilation_AIV2/1 -> Sum1/9
  THBr2/1 -> radiator2/2
  radiator2/2 -> THB_r2/1
  room_node_2/4 -> Ventilation_AIV2/4
  room_node_2/3 -> floor_in2/4
  Ground5/1 -> wall_out1/2
  Wall_in/2 -> Sum1/6
  air_exchange_rate/1 -> Ventilation_AIV1/1, Ventilation_AIV2/1
  room_node_1/1 -> wall with window1/2, wall with window2/2, ceiling1/3, floor_in1/1, radiator1/1, Ventilation_AIV1/2, Wall_in/1, wall_out/3, "[AIV]node1"/1
  room_node_2/1 -> wall_out1/3, floor_in2/1, radiator2/1, Ventilation_AIV2/2, ceiling2/3, Wall_in/3, wall with window4/2, wall with window3/2, "[AIV]node2"/1
  floor_in2/2 -> Terminator8/1  "T"
  floor_in1/2 -> Terminator5/1  "T"
  position4/1 -> floor_in1/2
  position6/1 -> floor_in2/2
  radiator1/1 -> Sum/10
  radiator2/1 -> Sum1/10
  Sum/1 -> room_node_1/1
  Sum1/1 -> room_node_2/1

== system carnot/Load/Houses/Simple_House ==
  WDB : Inport
  THB_in : Inport  Port=2
  Bus Creator : BusCreator  Inputs=5
  Bus Selector1 : BusSelector  OutputSignals=Temperature_Ambient
  Heattransfer2Ground_Simple : carnot/Load/Houses/heat_transfer/HeatTransfer2Ground_Simple  Tground=10  UAground=Uground*Floorsize(1)*Floorsize(2)
  House_OneNodeModel : carnot/Basic/Thermal_Models/House_OneNodeModel  Ahabit=Ahabit  Hroom=Hroom  tini=tini  UAout=UAwall  mc=mc  UAin=UAneighbour  dtroom=inf  AziWin=AziWin  Awin=Awin  Uwin=Uwin  Gwin=Gwin
  Radiator : carnot/Source/Heat_Exchanger/Radiator  pnom=heatload  dtnom=delta_t_nom  expo=n_rad  mcap=mass_times_cap  tini=tini  lin=0  qua=1000
  Ventilation : carnot/Source/Ventilation/Ventilation  vent=vent  rec=rec  Vhouse=Ahabit*Hroom
  const : Constant  Value=2.3
  const1 : Constant  Value=20
  shading : Relay  OnSwitchValue=24  OffSwitchValue=23  OnOutputValue=1-shade  OffOutputValue=1
  Hdat : Outport
  THB : Outport  Port=2
  wires:
  Ventilation/1 -> House_OneNodeModel/7
  const/1 -> House_OneNodeModel/4
  shading/1 -> House_OneNodeModel/6
  House_OneNodeModel/2 -> Bus Creator/2  "Qdot"
  const1/1 -> House_OneNodeModel/3
  Bus Creator/1 -> Hdat/1
  WDB/1 -> Bus Selector1/1, Bus Creator/5, House_OneNodeModel/1  "WDB"
  THB_in/1 -> Bus Creator/3, Radiator/2  "THB_in"
  House_OneNodeModel/1 -> Bus Creator/1, shading/1, Radiator/1, Ventilation/2, Heattransfer2Ground_Simple/1  "Troom"
  Radiator/2 -> Bus Creator/4, THB/1  "THB_out"
  Radiator/1 -> House_OneNodeModel/5  "Qdot"
  Heattransfer2Ground_Simple/1 -> House_OneNodeModel/2
  Bus Selector1/1 -> Ventilation/1  "<Temperature_Ambient>"

== system carnot/Load/Houses/Simple_House_ISO_GroundModel ==
  WDB : Inport
  THBin : Inport  Port=2
  Bus Creator : BusCreator  Inputs=5
  Bus Selector3 : BusSelector  OutputSignals=Temperature_Ambient
  Constant1 : Constant  Value=20
  House_OneNodeModel : carnot/Basic/Thermal_Models/House_OneNodeModel  Ahabit=Ahabit  Hroom=Hroom  tini=tini  UAout=UAwall  mc=mc  UAin=UAneighbour  dtroom=inf  AziWin=AziWin  Awin=Awin  Uwin=Uwin  Gwin=Gwin
  Internal_Gain_Profile : Subsystem
  Radiator : carnot/Source/Heat_Exchanger/Radiator  pnom=heatload  dtnom=delta_t_nom  expo=n_rad  mcap=mass_times_cap  tini=tini  lin=0  qua=1000
  Shading_Control : Subsystem
  Ventilation_Window : carnot/Source/Ventilation/Ventilation_Window  vent=vent  rec=rec  Vhouse=Ahabit*Hroom
  alfa_ground ISO13370_slabOnGround : carnot/Load/Houses/heat_transfer/HeatTransfer2Ground_ISO13370  wallsize=Floorsize  gammat=0  Tmeaninside=23.8  deltathetai=3.8  Tmeanoutside=11  deltathetae=9.3  tshift=319*3600  dwall=0.4  cond_ground=2.0  cp_ground=800  rho_ground=2500  rtot=1/Uground
  Hdat : Outport
  THBout : Outport  Port=2
  wires:
  WDB/1 -> Bus Selector3/1, Shading_Control/1(WDB), Bus Creator/5, House_OneNodeModel/1  "WDB"
  THBin/1 -> Radiator/2, Bus Creator/3  "THB_in"
  Radiator/2 -> THBout/1, Bus Creator/4  "THB_out"
  Ventilation_Window/1 -> House_OneNodeModel/7
  Constant1/1 -> House_OneNodeModel/3
  Radiator/1 -> House_OneNodeModel/5  "Qdot"
  Bus Selector3/1 -> Ventilation_Window/1  "<Temperature_Ambient>"
  House_OneNodeModel/1 -> Ventilation_Window/2, Shading_Control/2(Troom), Radiator/1, Bus Creator/1  "Troom"
  Shading_Control/1(Shading) -> House_OneNodeModel/6
  House_OneNodeModel/2 -> Bus Creator/2  "Qdot"
  Internal_Gain_Profile/1(Internal_Gain) -> House_OneNodeModel/4
  Bus Creator/1 -> Hdat/1
  alfa_ground ISO13370_slabOnGround/1 -> House_OneNodeModel/2

== system carnot/Load/Houses/Simple_House_ISOgm_CONF ==
  WDB : Inport
  THBin : Inport  Port=2
  Simple_House_ISO_GroundModel : carnot/Load/Houses/Simple_House_ISO_GroundModel  Ahabit=SH.Ahabit  Hroom=SH.Hroom  Floorsize=SH.Slab  UAwall=SH.UAwall  UAneighbour=0  Uground=0.2  mc=SH.cap  shade=SH.shading  tini=tini  Awin=SH.Awindow  AziWin=SH.AziWindow  Uwin=SH.Uwindow  Gwin=SH.Gwindow  vent=SH.Ventilationrate  rec=SH.Heatrecovery  heatload=SH.Heatload  delta_t_nom=SH.DTnomHeatingsystem  n_rad=SH.RadiatorExponent  mass_times_cap=SH.CapHeatingsystem  dpcoeff=SH.DpHeatingsystem
  Hdat : Outport
  THB : Outport  Port=2
  wires:
  WDB/1 -> Simple_House_ISO_GroundModel/1
  Simple_House_ISO_GroundModel/1 -> Hdat/1
  THBin/1 -> Simple_House_ISO_GroundModel/2
  Simple_House_ISO_GroundModel/2 -> THB/1

== system carnot/Load/Houses/heat_transfer ==
  HeatTransfer2Ground_ISO13370 : Subsystem  mask(Heat Transfer to Ground){wallsize=[7 10], gammat=0, Tmeaninside=23.8, deltathetai=3.8, Tmeanoutside=11, deltathetae=9.3, tshift=319*3600, dwall=0.4, cond_ground=2.0, cp_ground=800, rho_ground=2500, rtot=1./0.183}
      mask prompts: wallsize "size of slab [m] [length width]"; gammat "linear thermal transmittance associated with wall/floor junctions [W/mK]"; Tmeaninside "mean inside temperature over one year [°C]"; deltathetai "amplitude of monthly mean internal temperature [°C]"; Tmeanoutside "mean outside temperature over one year [°C]"; deltathetae "amplitude of monthly mean outside temperature [°C]"; tshift "time shift where external temperature sine-curve shows a mimimum [h]"; dwall "average thickness of side walls inlcuding all layers [m]"; cond_ground "conductivity of ground [W/(m*K)]"; cp_ground "capacity of ground [J/(kg*K)]"; rho_ground "density of ground [kg/m^3]"; rtot "total thermal resistance of slab (between Troom and Tground) [m²K/W]"
      mask help: Ground heat transfer for a floor "SLAB ON GROUND" according to ISO 13370:2007.
  HeatTransfer2Ground_Simple : Subsystem  mask(Heat Transfer to Ground simple Model){Tground=10, UAground=0.2*70}
      mask prompts: Tground "Ground temperature in °C"; UAground "Heat transfer to ground in W/K"
  alfa_ceiling : Subsystem  mask(ALFA){active=0, emission_c=0.65, wallsurface=1}
      mask prompts: active "active layer (0 / 1)"; emission_c "Longwave emissivity of surface (0..1)"; wallsurface "Ceiling surface in m²"
      mask help:
      | Convective and radiative heat transfer at the SURFACE OF A HORIZONTAL CEELING.
      | [AIV] : conditions of zone node,
      | Ts : temperature of outdoor wall surface, °C,
      | qdots : specific heat flow into wall construction, W/m^2,
      | [S] : heat and air flow to zone node.
  alfa_floor : Subsystem  mask(ALFA){active=0, emission_f=0.65, wallsurface=1}
      mask prompts: active "active layer (0 / 1)"; emission_f "Longwave emissivity of surface (0..1)"; wallsurface "Floor surface in m²"
      mask help:
      | Convective and radiative heat transfer at the SURFACE OF A HORIZONTAL FLOOR.
      |
      | [AIV] : conditions of zone node,
      | Ts : temperature of wall surface, °C,
      | qdots : specific heat flow into wall construction, W/m^2,
      | [S] : heat and air flow to zone node.
  alfa_wall_in : Subsystem  mask(ALFA){active=0, emission_in=0.7, wallsurface=1}
      mask prompts: active "Active layer (0 / 1)"; emission_in "Longwave emissivity of surface (0..1)"; wallsurface "Wall surface in m²"
      mask help:
      | Convective and radiative heat transfer at the INDOOR SURFACE of a VERTICAL OUTER WALL.
      |
      | [AIV] : conditions of zone node,
      | Ts : temperature of wall surface, °C,
      | qdots : specific heat flow into wall construction, W/m^2,
      | [S] : heat and air flow to zone node.
  alfa_wall_out : Subsystem  mask(ALFA){pos=0, absorption_out=0.4, emission_out=0.7, wallsurface=1}
      mask prompts: pos "Azimut (south = 0, east = -90) in degrees"; absorption_out "Solar absorption outside (0..1)"; emission_out "Longwave emissivity of surface (0..1)"; wallsurface "Wall surface in m²"
      mask help:
      | Convective and radiative HEAT TRANSFER at the WEATHER EXPOSED SURFACE of an OUTER WALL.
      |
      | [W*] : modified weather data, adapted to height over ground,
      | Ts : temperature of outdoor wall surface, °C,
      | qdots : specific heat flow into wall / window construction, W/m^2.
      mask init:
      | if length(pos) == 1
      |     pos = [90  pos 0]; % pos is [inclination azimut rotation]
      | end
  alfa_window_in : Subsystem  mask(ALFA){gvalue=0.7, emission_in=0.87, wallsurface=1, frame=0.1, numlayer=2}
      mask prompts: gvalue "Energy transmission by sunlight (g-value) 0..1"; emission_in "Longwave emissivity (0..1)"; wallsurface "Surface of the window (with frame) in m²"; frame "Share of the frame on the surface (0...1)"; numlayer "Number of glass panes"
      mask help:
      | Convective and radiative heat transfer at the INDOOR SURFACE OF A VERTICAL WINDOW with 1-4 layers (each 3 ... 8 mm thick).
      |
      | Ts  : temperature of window surface, °C,
      | [sun_t]  : sun data (incidence angle, direct and diffuse radiation
      |     at tilted window surface),
      | [AIV]  : conditions of zone node,
      | qdots  : specific heat flow into window construction, W/m^2,
      | qdot_abs : specific irradiation absorption within window
      |     construction,  W/m^2,
      | [S]  : heat and air flow to zone node.
  alfa_window_out : Subsystem  mask(ALFA){pos=0, absorption_out=0.01, emission_out=0.87, frame=0.1}
      mask prompts: pos "Azimut of the surface (South = 0; East = -90)"; absorption_out "Solar absorption of the glass (0...1)"; emission_out "Longwave emissivity (0...1)"; frame "Share of the frame on the surface (0..1)"
      mask help:
      | Convective and radiative heat transfer at the OUTDOOR SURFACE OF A VERTICAL WINDOW.
      | Azimut can be a scalar or a vector with [inclination azimut rotation].
      | [W*] : modified weather data, adapted to height over ground,
      | Ts : temperature of outdoor window surface, °C,
      | qdots : specific heat flow into window construction, W/m^2,
      | [sun_t] : sun data (incidence angle, direct and diffuse radiation
      |                  at tilted window surface).
      mask init:
      | if length(pos) == 1
      |     pos = [90  pos 0]; % pos is [inclination azimut rotation]
      | end
  wall_out_IR_radiation : Subsystem

== system carnot/Load/Houses/room_nodes ==
  Room_Node : Subsystem  mask(NODE){zoneairvolume=5*5*2.5, zoneheight=2.5, zonestartTEMP=20, zonestartWATER=55, timeconst=100, heatperfect=natural, lookuptime=[0 24]*3600, lookupvalue=[20 20], AirPressure=101300}
      mask prompts: zoneairvolume "SIZE: netto air volume >0, m^3"; zoneheight "SIZE: height of zone (floor - ceiling) >0, m"; zonestartTEMP "START TEMPERATURE: convective and radiative node, °C"; zonestartWATER "START AIR HUMIDITY: relative air humidity [0,100], %"; timeconst "timeconstant of radiative and convective node in s"; heatperfect "air temperature"; lookuptime "time vector for ideal profile [s]"; lookupvalue "values for ideal profile [degree centigrade]"; AirPressure "Air pressure for material properties in Pa"
      mask help:
      | This block delivers the energy consumption, temperature and air quality of a zone.
      | It is assumed that this node represents the center of a zone all connected sink and source blocks communicate with. Sink and source blocks are walls, windows, persons, heater etc..
      | Properties of air are calculated once at initialization (with node start temperature, humidity and air pressure).
      | [S] : input vector from sink blocks and source blocks
      | [AIV] : output vector with node temperature and air quality data.
      mask init:
      | CO2norm = 400*1e-6;
      | zoneairvolume = max(0.01, zoneairvolume);
      | zoneheight = max(0.01, zoneheight);
      | zonestartWATER = min(100, max(0, zonestartWATER));
      | zonestartWATER = rel_hum2x(zonestartTEMP, 10^5, zonestartWATER)*1.18*zoneairvolume; % kg H2O in zone volume (at 20°C)
      | zonestartCO2 = CO2norm*1.529*zoneairvolume; % kg CO2 in zone volume
      | zonestartAIR = 10^5*zoneairvolume/(287*(zonestartTEMP+273)); % kg AIR in zone volume
      mask Help: web(fullfile(path_carnot('help'),'Room_Node.html'),'-helpbrowser')
      mask TypeOptions heatperfect: natural | ideal profile (for heating demand)

== system carnot/Load/Houses/ventilation_heating ==
  Floorheating_TABS : Subsystem  mask(FBH-TABS){d=0.08, d1=0.04, d_pipe=0.016, dr=0.002, dx=0.1, l=700, lambda_r=0.35, lambda_b=1.4}
      mask prompts: d "thickness of active layer [m]"; d1 "depth of pipes in active layer [m]"; d_pipe "outer diameter of pipes [m]"; dr "wall thickness of pipe [m]"; dx "distance between center of pipes [m]"; l "length of pipe [m]"; lambda_r "conductivity of pipe [W/(m*K)]"; lambda_b "conductivity of layer material [W/(m*K)]"
      mask help:
      | calculates the heating/cooling power from pipes
      | in a floor heating system or a thermally active building component
      | to the active layer in the building element (wall, floor, ceiling)
      | according to the model of M.Koschenz & B.Lehmann, EMPA-CH, 2000
  THB_P_adapter : Subsystem  mask(ACTIVE COMPONENT){mass=1, ua=800*5*5/0.2*0.022*3.1415, t0=20}
      mask prompts: mass "MASS of fluid in heating element >0, kg"; ua "HEAT TRANSFER of fluid <-> wall >0, W/K"; t0 "start temperature in °C"
      mask help:
      | Adapter between active components and house-model.
      |
      | Transformation from heat flow - defined by the thermo-hydraulic vector THV - to an "electric" power entering the block "active wall", "active ceiling", "active floor" or "flat radiator".
      |
      | P  : "electric" power flowing into active layer of wall, W
      | T(P)  : temperature of active layer, °C
      | THV_in  : hydraulic vector input
      | THV_out : hydraulic vector output
      mask init:
      | mass = str2num(mass);
      | if length(mass)~=1 error(['PARAMETERS block "' path2block '" : "MASS ..." must have only 1 entry !']); end;
      | if (mass<=0) error(['PARAMETERS block "' path2block '" : "MASS ..." must be >0 !']); end;
      | 
      | ua = str2num(ua);
      | if length(ua)~=1 error(['PARAMETERS block "' path2block '" : "HEAT TRANSFER ..." must have only 1 entry !']); end;
      | if (ua<=0) error(['PARAMETERS block "' path2block '" : "HEAT TRANSFER ..." must be >0 !']); end;
      mask Help: eval('man (''THV_P_adapter'')')
  Ventilation : carnot/Source/Ventilation/Ventilation  vent=vent  rec=rec  Vhouse=Ahabit*Hroom
  Ventilation_AIV : carnot/Source/Ventilation/Ventilation_AIV  co2=400
  Ventilation_Window : carnot/Source/Ventilation/Ventilation_Window  vent=vent  rec=rec  Vhouse=Ahabit*Hroom
